simulink model "flight_sim"  (R2024b)
settings: Solver=VariableStepAuto  StartTime=0.0  StopTime=10.0  RelTol=1e-3
model workspace: external: MAT-File C:\Users\filip\OneDrive - VUT\ING_4.semestr\CPSa\Project\My\fdm.mat (data not in the file)
values from neighbouring files (symbols this model uses):
  lat_A = lat_C' * lat_A_pre    [fdm.m]
  lat_B = lat_C' * lat_B_pre    [fdm.m]
  lon_A = lon_C' * lon_A_pre    [fdm.m]
  lon_B = lon_C' * lon_B_pre    [fdm.m]
  P_s = 0    [fdm.m]
  phi_s = 0    [fdm.m]
  psi_s = 0    [fdm.m]
  Q_s = 0    [fdm.m]
  R_s = 0    [fdm.m]
  theta_s = 0    [fdm.m]
  V_TAS_s = 205.13    [fdm.m]
undefined symbols (not defined in the file or in its folder): Earth, WGS84
libraries: aerolibfltsims x2, shared6dof x1, aerolibtransform2 x1
settings Model: Creator=sara  LastModifiedBy=filip

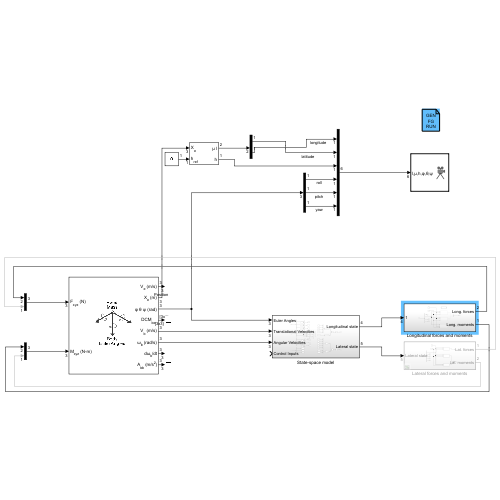
[thumbnail: Simulink's stored preview of the top-level diagram]
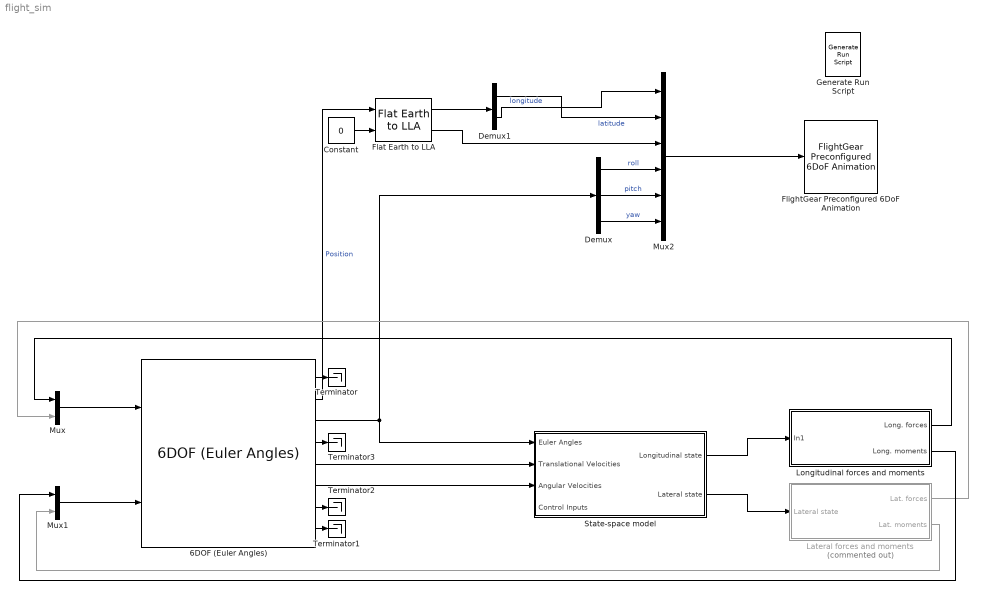
== system flight_sim ==
  6DOF (Euler Angles) : shared6dof/6DOF (Euler Angles)  units=Metric (MKS)  mtype=Fixed  rep=Euler Angles  xme_0=[0 0 0]  Vm_0=[0 0 0]  eul_0=[0 0 0]  pm_0=[0 0 0]  mass_0=1.0  mass_e=0.5  mass_f=2.0  inertia=eye(3)  inertia_e=eye(3)  inertia_f=2*eye(3)  k_quat=1.0  vre_flag=on  abi_flag=off  aMode=0  xme_statename=''  Vm_statename=''  eul_statename=''  quat_statename=''  pm_statename=''  mass_statename=''
  Constant : Constant  Value=0
  Demux : Demux  Outputs=3
  Demux1 : Demux  Outputs=2
  Flat Earth to LLA : aerolibtransform2/Flat Earth to LLA  units=Metric (MKS)  ptype=Earth (WGS84)  F=1/298.257223563  R=6378137  refPosPort=off  LL0=[0 10]  psi=0
  FlightGear Preconfigured 6DoF Animation : aerolibfltsims/FlightGear Preconfigured 6DoF Animation  xFlightGearVersion=v2019.1  DestinationIpAddress=127.0.0.1  DestinationPort=5502  SampleTime=1/30  packetVersion=24
  Generate Run Script : aerolibfltsims/Generate Run Script  Architecture=Default  dataFlow=Send  GeometryModelName=HL20  AirportId=KSFO  RunwayId=10L  InitialAltitude=7224  InitialHeading=113  OffsetDistance=4.72  OffsetAzimuth=0  InstallScenery=off  DisableShaders=off  OriginAddress=127.0.0.1  DestinationPort=5502  OriginPort=5505  LocalAddress=127.0.0.1  OutputFileName=runfg.bat  FlightGearBaseDirectory=C:\Program Files\FlightGear
  Lateral forces and moments : Subsystem  Commented=on
  Longitudinal forces and moments : Subsystem
  Mux : Mux  Inputs=2
  Mux1 : Mux  Inputs=2
  Mux2 : Mux  Inputs=6
  State-space model : Subsystem
  Terminator{,1..3} (4 alike) : Terminator
  wires:
  6DOF (Euler Angles)/1 -> Terminator/1
  6DOF (Euler Angles)/5 -> State-space model/2(Translational Velocities)
  6DOF (Euler Angles)/6 -> State-space model/3(Angular Velocities)
  6DOF (Euler Angles)/3 -> Demux/1, State-space model/1(Euler Angles)
  6DOF (Euler Angles)/8 -> Terminator1/1
  6DOF (Euler Angles)/7 -> Terminator2/1
  6DOF (Euler Angles)/2 -> Flat Earth to LLA/1  "Position"
  6DOF (Euler Angles)/4 -> Terminator3/1
  State-space model/1(Longitudinal state) -> Longitudinal forces and moments/1(In1)
  State-space model/2(Lateral state) -> Lateral forces and moments/1(Lateral state)
  Mux/1 -> 6DOF (Euler Angles)/1
  Mux1/1 -> 6DOF (Euler Angles)/2
  Longitudinal forces and moments/1(Long. forces) -> Mux/1
  Lateral forces and moments/1(Lat. forces) -> Mux/2
  Lateral forces and moments/2(Lat. moments) -> Mux1/2
  Longitudinal forces and moments/2(Long. moments) -> Mux1/1
  Mux2/1 -> FlightGear Preconfigured 6DoF Animation/1
  Demux/3 -> Mux2/6  "yaw"
  Demux/2 -> Mux2/5  "pitch"
  Demux/1 -> Mux2/4  "roll"
  Demux1/1 -> Mux2/2  "latitude"
  Demux1/2 -> Mux2/1  "longitude"
  Flat Earth to LLA/1 -> Demux1/1
  Flat Earth to LLA/2 -> Mux2/3
  Constant/1 -> Flat Earth to LLA/2

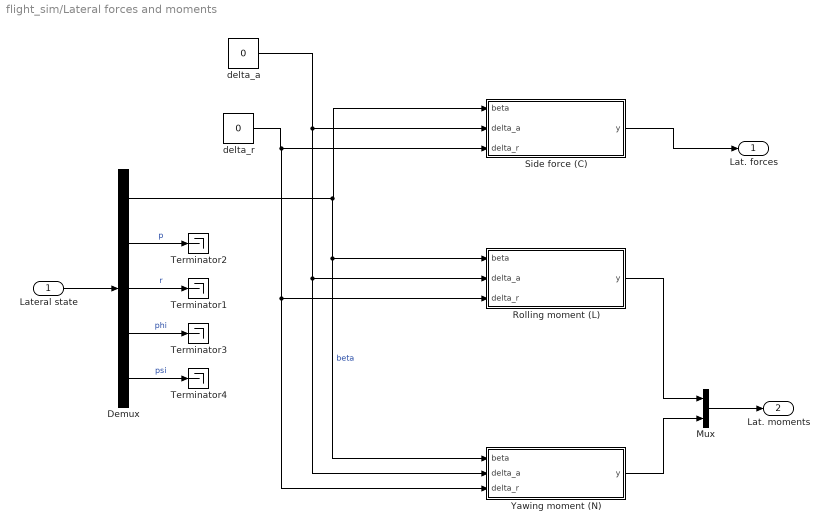
== system flight_sim/Lateral forces and moments ==
  Lateral state : Inport
  Demux : Demux  Outputs=5
  Mux : Mux  Inputs=2
  Rolling moment (L) : MATLAB Function  TreatAsAtomicUnit=on
  Side force (C) : MATLAB Function  TreatAsAtomicUnit=on
  Terminator{1..4} (4 alike) : Terminator
  Yawing moment (N) : MATLAB Function  TreatAsAtomicUnit=on
  delta_a : Constant  Value=0
  delta_r : Constant  Value=0
  Lat. forces : Outport
  Lat. moments : Outport  Port=2
  wires:
  Lateral state/1 -> Demux/1
  Demux/1 -> Yawing moment (N)/1(beta), Rolling moment (L)/1(beta), Side force (C)/1(beta)  "beta"
  Demux/2 -> Terminator2/1  "p"
  Demux/3 -> Terminator1/1  "r"
  Demux/4 -> Terminator3/1  "phi"
  Demux/5 -> Terminator4/1  "psi"
  Side force (C)/1(y) -> Lat. forces/1
  delta_a/1 -> Yawing moment (N)/2(delta_a), Rolling moment (L)/2(delta_a), Side force (C)/2(delta_a)
  delta_r/1 -> Rolling moment (L)/3(delta_r), Yawing moment (N)/3(delta_r), Side force (C)/3(delta_r)
  Mux/1 -> Lat. moments/1
  Rolling moment (L)/1(y) -> Mux/1
  Yawing moment (N)/1(y) -> Mux/2

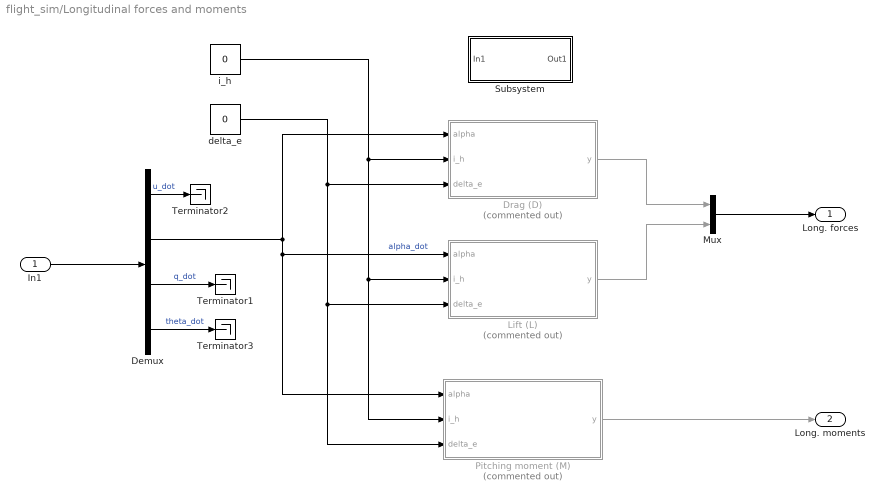
== system flight_sim/Longitudinal forces and moments ==
  In1 : Inport
  Demux : Demux
  Drag (D) : MATLAB Function  Commented=on  TreatAsAtomicUnit=on
  Lift (L) : MATLAB Function  Commented=on  TreatAsAtomicUnit=on
  Mux : Mux  Inputs=2
  Pitching moment (M) : MATLAB Function  Commented=on  TreatAsAtomicUnit=on
  Subsystem : Subsystem
  Terminator1 : Terminator
  Terminator2 : Terminator
  Terminator3 : Terminator
  delta_e : Constant  Value=0
  i_h : Constant  Value=0
  Long. forces : Outport
  Long. moments : Outport  Port=2
  wires:
  In1/1 -> Demux/1
  Demux/1 -> Terminator2/1  "u_dot"
  Demux/2 -> Pitching moment (M)/1(alpha), Lift (L)/1(alpha), Drag (D)/1(alpha)  "alpha_dot"
  Demux/3 -> Terminator1/1  "q_dot"
  Demux/4 -> Terminator3/1  "theta_dot"
  i_h/1 -> Pitching moment (M)/2(i_h), Lift (L)/2(i_h), Drag (D)/2(i_h)
  delta_e/1 -> Drag (D)/3(delta_e), Pitching moment (M)/3(delta_e), Lift (L)/3(delta_e)
  Drag (D)/1(y) -> Mux/1
  Mux/1 -> Long. forces/1
  Lift (L)/1(y) -> Mux/2
  Pitching moment (M)/1(y) -> Long. moments/1

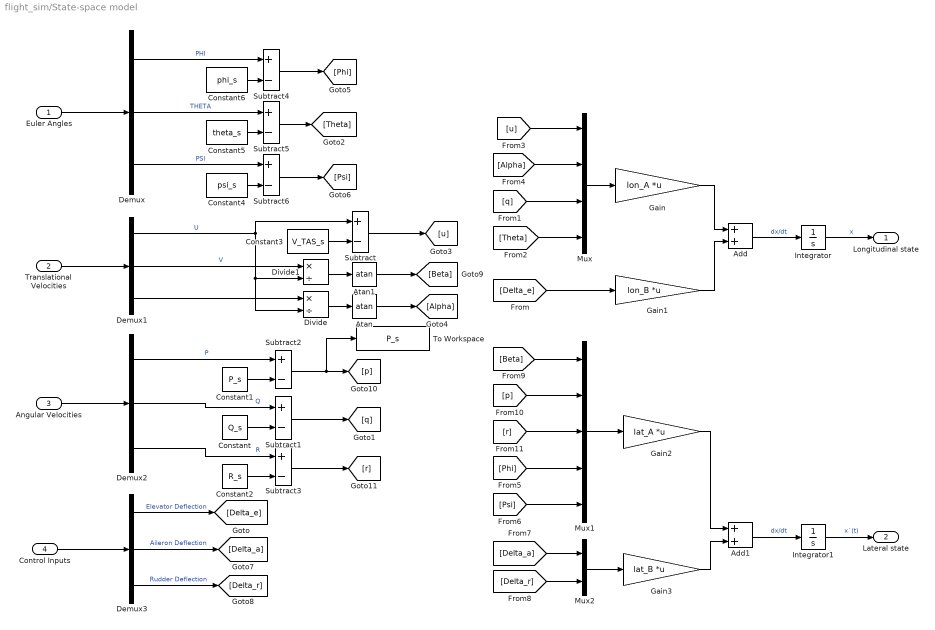
== system flight_sim/State-space model ==
  Euler Angles : Inport
  Translational Velocities : Inport  Port=2
  Angular Velocities : Inport  Port=3
  Control Inputs : Inport  Port=4
  Add : Sum
  Add1 : Sum
  Atan : Trigonometry  Operator=atan
  Atan1 : Trigonometry  Operator=atan
  Constant : Constant  Value=Q_s
  Constant1 : Constant  Value=P_s
  Constant2 : Constant  Value=R_s
  Constant3 : Constant  Value=V_TAS_s
  Constant4 : Constant  Value=psi_s
  Constant5 : Constant  Value=theta_s
  Constant6 : Constant  Value=phi_s
  Demux{,1..3} (4 alike) : Demux  Outputs=3
  Divide : Product  Inputs=*/
  Divide1 : Product  Inputs=*/
  Gain : Gain  Gain=lon_A  Multiplication=Matrix(K*u)
  Gain1 : Gain  Gain=lon_B  Multiplication=Matrix(K*u)
  Gain2 : Gain  Gain=lat_A  Multiplication=Matrix(K*u)
  Gain3 : Gain  Gain=lat_B  Multiplication=Matrix(K*u)
  Integrator : Integrator
  Integrator1 : Integrator
  Mux : Mux
  Mux1 : Mux  Inputs=5
  Mux2 : Mux  Inputs=2
  Subtract{,1..6} (7 alike) : Sum  Inputs=+-
  To Workspace : ToWorkspace  VariableName=P_s  SaveFormat=Timeseries  SampleTime=-1
  Longitudinal state : Outport
  Lateral state : Outport  Port=2
  wires:
  Demux1/2 -> Divide1/1  "V"
  Euler Angles/1 -> Demux/1
  Translational Velocities/1 -> Demux1/1
  Demux2/3 -> Subtract3/1  "R"
  Demux2/1 -> Subtract2/1  "P"
  Angular Velocities/1 -> Demux2/1
  Gain/1 -> Add/1
  Add/1 -> Integrator/1  "dx/dt"
  Demux1/3 -> Divide/1
  Gain1/1 -> Add/2
  Demux2/2 -> Subtract1/1  "Q"
  Demux1/1 -> Subtract/1, Divide1/2, Divide/2  "U"
  Demux3/1 -> [Delta_e]  "Elevator Deflection"
  Divide/1 -> Atan/1
  Mux/1 -> Gain/1
  Control Inputs/1 -> Demux3/1
  Demux3/2 -> [Delta_a]  "Aileron Deflection"
  Demux3/3 -> [Delta_r]  "Rudder Deflection"
  Integrator/1 -> Longitudinal state/1  "x"
  [Delta_e] -> Gain1/1
  Subtract1/1 -> [q]
  [q] -> Mux/3
  [Theta] -> Mux/4
  Subtract/1 -> [u]
  [u] -> Mux/1
  Atan/1 -> [Alpha]
  [Alpha] -> Mux/2
  Mux2/1 -> Gain3/1
  Mux1/1 -> Gain2/1
  Add1/1 -> Integrator1/1  "dx/dt"
  Integrator1/1 -> Lateral state/1  "x˙(t)"
  Gain3/1 -> Add1/2
  Gain2/1 -> Add1/1
  [Phi] -> Mux1/4
  [Psi] -> Mux1/5
  [Delta_a] -> Mux2/1
  [Delta_r] -> Mux2/2
  Atan1/1 -> [Beta]
  Divide1/1 -> Atan1/1
  [Beta] -> Mux1/1
  Subtract2/1 -> To Workspace/1, [p]
  Subtract3/1 -> [r]
  Constant2/1 -> Subtract3/2
  [p] -> Mux1/2
  [r] -> Mux1/3
  Constant6/1 -> Subtract4/2
  Subtract4/1 -> [Phi]
  Demux/1 -> Subtract4/1  "PHI"
  Constant5/1 -> Subtract5/2
  Subtract5/1 -> [Theta]
  Demux/2 -> Subtract5/1  "THETA"
  Constant4/1 -> Subtract6/2
  Subtract6/1 -> [Psi]
  Demux/3 -> Subtract6/1  "PSI"
  Constant3/1 -> Subtract/2
  Constant/1 -> Subtract1/2
  Constant1/1 -> Subtract2/2

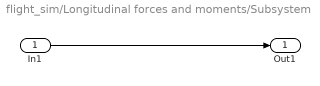
== system flight_sim/Longitudinal forces and moments/Subsystem ==
  In1 : Inport
  Out1 : Outport
  wires:
  In1/1 -> Out1/1

== matlab function flight_sim/Longitudinal forces and moments/Lift (L) ==
  data: alpha input; y output; i_h input; delta_e input
function y = fcn(alpha, i_h, delta_e)
    y = (C_L0 + C_Lalpha * alpha + C_lih * i_h + C_ldelta_e * delta_e) * q_bar * S;

== matlab function flight_sim/Longitudinal forces and moments/Drag (D) ==
  data: y output; alpha input; i_h input; delta_e input
function y = fcn(alpha, i_h, delta_e)
    y = (C_D0 + C_Dalpha * alpha + C_dih * i_h + C_ddelta_e * delta_e) * q_bar * S;

== matlab function flight_sim/Longitudinal forces and moments/Pitching moment (M) ==
  data: alpha input; y output; i_h input; delta_e input
function y = fcn(alpha, i_h, delta_e)
    coder.extrinsic('evalin'); % Allows using base workspace variables
    C_m0 = evalin('base', 'C_m0'); 
    C_malpha = evalin('base', 'C_malpha'); 
    C_mih = evalin('base', 'C_mih'); 
    C_mdelta_e = evalin('base', 'C_mdelta_e'); 
    q_bar = evalin('base', 'q_bar'); 
    S = evalin('base', 'S'); 
    c_bar = evalin('base', 'c_bar'); 
    y = (C_m0 + C_malpha * alpha + C_mih * i_h + C_mdelta_e * delta_e) * q_bar * S * c_bar;

== matlab function flight_sim/Lateral forces and moments/Side force (C) ==
  data: beta input; y output; delta_a input; delta_r input
function y = fcn(beta, delta_a, delta_r)
    coder.extrinsic('evalin'); % Allows using base workspace variables
    C_y0 = evalin('base', 'C_y0'); 
    C_ybeta = evalin('base', 'C_ybeta'); 
    C_ydelta_a = evalin('base', 'C_ydelta_a'); 
    C_ydelta_r = evalin('base', 'C_ydelta_r'); 
    q_bar = evalin('base', 'q_bar'); 
    S = evalin('base', 'S'); 
    y = (C_y0 + C_ybeta * beta + C_ydelta_a * delta_a + C_ydelta_r * delta_r) * q_bar * S;

== matlab function flight_sim/Lateral forces and moments/Rolling moment (L) ==
  data: beta input; y output; delta_a input; delta_r input
function y = fcn(beta, delta_a, delta_r)
    coder.extrinsic('evalin'); % Allows using base workspace variables
    C_L0 = evalin('base', 'C_L0'); 
    C_lbeta = evalin('base', 'C_lbeta'); 
    C_ldelta_a = evalin('base', 'C_ldelta_a'); 
    C_ldelta_r = evalin('base', 'C_ldelta_r'); 
    q_bar = evalin('base', 'q_bar'); 
    S = evalin('base', 'S'); 
    b = evalin('base', 'b'); 
    y = (C_L0 + C_lbeta * beta + C_ldelta_a * delta_a + C_ldelta_r * delta_r) * q_bar * S * b;

== matlab function flight_sim/Lateral forces and moments/Yawing moment (N) ==
  data: beta input; y output; delta_a input; delta_r input
function y = fcn(beta, delta_a, delta_r)
    coder.extrinsic('evalin'); % Allows using base workspace variables
    C_n0 = evalin('base', 'C_n0'); 
    C_nbeta = evalin('base', 'C_nbeta'); 
    C_ndelta_a = evalin('base', 'C_ndelta_a'); 
    C_ndelta_r = evalin('base', 'C_ndelta_r'); 
    q_bar = evalin('base', 'q_bar'); 
    S = evalin('base', 'S'); 
    b = evalin('base', 'b'); 
    y = (C_n0 + C_nbeta * beta + C_ndelta_a * delta_a + C_ndelta_r * delta_r) * q_bar * S * b;
